simulink model "Tarea_3"  (R2013a)
settings: Solver=ode23  StartTime=0.0  StopTime=10.0  RelTol=1e-3
settings Model: Creator=Miguel  LastModifiedBy=Miguel

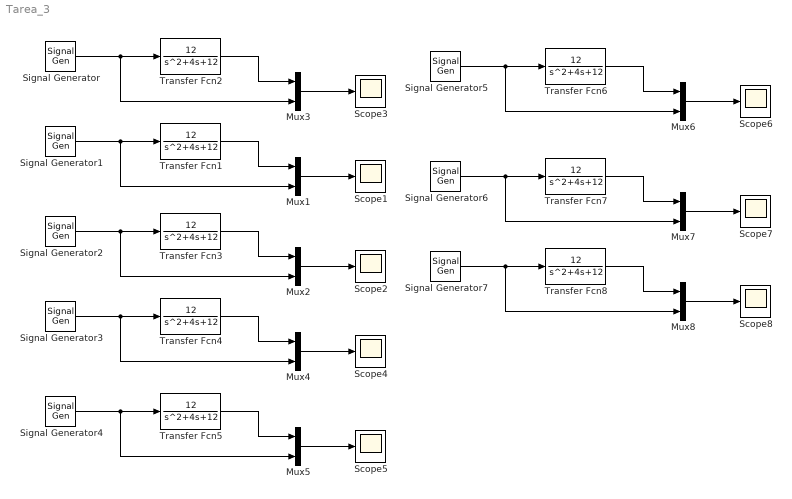
== system Tarea_3 ==
  Mux{1..8} (8 alike) : Mux  Inputs=2
  Scope{1..8} (8 alike) : Scope
      Scope1 settings: ShowLegends=on
      Scope2 settings: ShowLegends=on  SaveName=ScopeData2
      Scope3 settings: ShowLegends=on
      Scope4 settings: ShowLegends=on  SaveName=ScopeData3
      Scope5 settings: ShowLegends=on  SaveName=ScopeData4
      Scope6 settings: ShowLegends=on  SaveName=ScopeData5
      Scope7 settings: ShowLegends=on  SaveName=ScopeData6
      Scope8 settings: ShowLegends=on  SaveName=ScopeData7
  Signal Generator : SignalGenerator
  Signal Generator1 : SignalGenerator  Units=rad/sec
  Signal Generator2 : SignalGenerator  WaveForm=square
  Signal Generator3 : SignalGenerator  WaveForm=sawtooth  Units=rad/sec
  Signal Generator4 : SignalGenerator  WaveForm=random  Units=rad/sec
  Signal Generator5 : SignalGenerator  WaveForm=random  Amplitude=2  Frequency=3
  Signal Generator6 : SignalGenerator  Amplitude=2  Frequency=10
  Signal Generator7 : SignalGenerator  Amplitude=4  Frequency=10
  Transfer Fcn{1..8} (8 alike) : TransferFcn  Numerator=[12]  Denominator=[1 4 12]
  wires:
  Transfer Fcn2/1 -> Mux3/1
  Signal Generator/1 -> Mux3/2, Transfer Fcn2/1
  Mux3/1 -> Scope3/1
  Transfer Fcn1/1 -> Mux1/1
  Signal Generator1/1 -> Mux1/2, Transfer Fcn1/1
  Mux1/1 -> Scope1/1
  Transfer Fcn3/1 -> Mux2/1
  Signal Generator2/1 -> Mux2/2, Transfer Fcn3/1
  Mux2/1 -> Scope2/1
  Transfer Fcn4/1 -> Mux4/1
  Signal Generator3/1 -> Mux4/2, Transfer Fcn4/1
  Mux4/1 -> Scope4/1
  Transfer Fcn5/1 -> Mux5/1
  Signal Generator4/1 -> Mux5/2, Transfer Fcn5/1
  Mux5/1 -> Scope5/1
  Transfer Fcn6/1 -> Mux6/1
  Signal Generator5/1 -> Mux6/2, Transfer Fcn6/1
  Mux6/1 -> Scope6/1
  Transfer Fcn7/1 -> Mux7/1
  Signal Generator6/1 -> Mux7/2, Transfer Fcn7/1
  Mux7/1 -> Scope7/1
  Transfer Fcn8/1 -> Mux8/1
  Signal Generator7/1 -> Mux8/2, Transfer Fcn8/1
  Mux8/1 -> Scope8/1
